simulink model "CODRTIV_v2_SystemContext"  (R2026a)
settings: Solver=VariableStepAuto
settings Model: Creator=pwilliam  LastModifiedBy=pwilliam

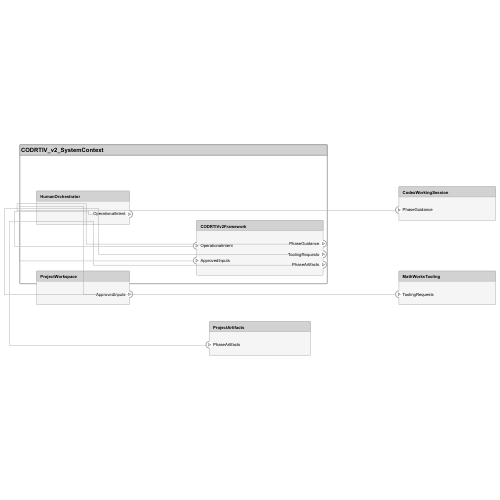
[thumbnail: Simulink's stored preview of the top-level diagram]
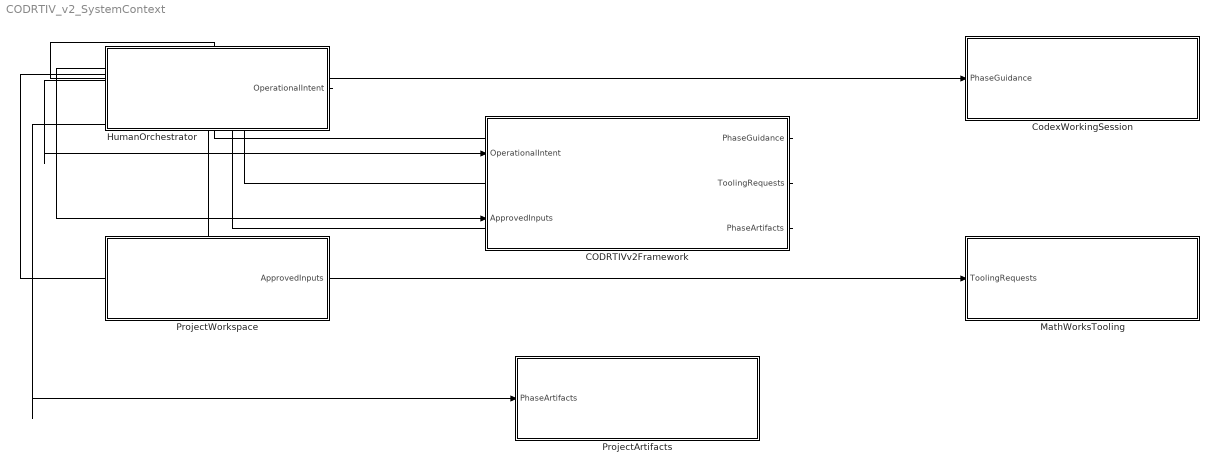
== system CODRTIV_v2_SystemContext ==
  CODRTIVv2Framework : Subsystem
      settings: PortSchema="{\"entries\":[{\"content\":{\"headerSize\":26,\"margin\":15,\"minimumSpacing\":25,\"sides\":[{\"content\":{\"connectorIds\":[\"In1\",\"In2\"]},\"type\":\"ConnectorPlacement.EquallySpacedRectSide\",\"uuid\":\"d8a99cda-410f-444c-a2c0-34a0f9144019\"},{\"content\":{\"connectorIds\":[\"Out1\",\"Out2\",\"Out3\"],\"side\":\"RIGHT\"},\"type\":\"ConnectorPlacement.EquallySpacedRectSide\",\"uuid\":\"6fbfd3a0-bc9b-423f-a970-aec3e1e13485\"},{\"content\":{\"side\":\"TOP\"},\"type\":\"ConnectorPlacement.EquallySpacedRectSide\",\"uuid\":\"0cbf1f34-d469-4804-b698-a8f91b09beec\"}]},\"type\":\"ConnectorPlacement.EquallySpacedConnector\",\"uuid\":\"a084b8e2-295c-4f11-89a7-efdb21efd295\"}],\"packageUris\":[\"http://schema.mathworks.com/mf0/Connector/R2020b\"],\"version\":\"1.0\"}"
  CodexWorkingSession : Subsystem
      settings: PortSchema="{\"entries\":[{\"content\":{\"headerSize\":26,\"margin\":15,\"minimumSpacing\":25,\"sides\":[{\"content\":{\"connectorIds\":[\"In1\"]},\"type\":\"ConnectorPlacement.EquallySpacedRectSide\",\"uuid\":\"d8a99cda-410f-444c-a2c0-34a0f9144019\"},{\"content\":{\"side\":\"RIGHT\"},\"type\":\"ConnectorPlacement.EquallySpacedRectSide\",\"uuid\":\"6fbfd3a0-bc9b-423f-a970-aec3e1e13485\"},{\"content\":{\"side\":\"TOP\"},\"type\":\"ConnectorPlacement.EquallySpacedRectSide\",\"uuid\":\"0cbf1f34-d469-4804-b698-a8f91b09beec\"}]},\"type\":\"ConnectorPlacement.EquallySpacedConnector\",\"uuid\":\"a084b8e2-295c-4f11-89a7-efdb21efd295\"}],\"packageUris\":[\"http://schema.mathworks.com/mf0/Connector/R2020b\"],\"version\":\"1.0\"}"
  HumanOrchestrator : Subsystem
      settings: PortSchema="{\"entries\":[{\"content\":{\"headerSize\":26,\"margin\":15,\"minimumSpacing\":25,\"sides\":[{\"content\":{},\"type\":\"ConnectorPlacement.EquallySpacedRectSide\",\"uuid\":\"d8a99cda-410f-444c-a2c0-34a0f9144019\"},{\"content\":{\"connectorIds\":[\"Out1\"],\"side\":\"RIGHT\"},\"type\":\"ConnectorPlacement.EquallySpacedRectSide\",\"uuid\":\"6fbfd3a0-bc9b-423f-a970-aec3e1e13485\"},{\"content\":{\"side\":\"TOP\"},\"type\":\"ConnectorPlacement.EquallySpacedRectSide\",\"uuid\":\"0cbf1f34-d469-4804-b698-a8f91b09beec\"}]},\"type\":\"ConnectorPlacement.EquallySpacedConnector\",\"uuid\":\"a084b8e2-295c-4f11-89a7-efdb21efd295\"}],\"packageUris\":[\"http://schema.mathworks.com/mf0/Connector/R2020b\"],\"version\":\"1.0\"}"
  MathWorksTooling : Subsystem
      settings: PortSchema="{\"entries\":[{\"content\":{\"headerSize\":26,\"margin\":15,\"minimumSpacing\":25,\"sides\":[{\"content\":{\"connectorIds\":[\"In1\"]},\"type\":\"ConnectorPlacement.EquallySpacedRectSide\",\"uuid\":\"d8a99cda-410f-444c-a2c0-34a0f9144019\"},{\"content\":{\"side\":\"RIGHT\"},\"type\":\"ConnectorPlacement.EquallySpacedRectSide\",\"uuid\":\"6fbfd3a0-bc9b-423f-a970-aec3e1e13485\"},{\"content\":{\"side\":\"TOP\"},\"type\":\"ConnectorPlacement.EquallySpacedRectSide\",\"uuid\":\"0cbf1f34-d469-4804-b698-a8f91b09beec\"}]},\"type\":\"ConnectorPlacement.EquallySpacedConnector\",\"uuid\":\"a084b8e2-295c-4f11-89a7-efdb21efd295\"}],\"packageUris\":[\"http://schema.mathworks.com/mf0/Connector/R2020b\"],\"version\":\"1.0\"}"
  ProjectArtifacts : Subsystem
      settings: PortSchema="{\"entries\":[{\"content\":{\"headerSize\":26,\"margin\":15,\"minimumSpacing\":25,\"sides\":[{\"content\":{\"connectorIds\":[\"In1\"]},\"type\":\"ConnectorPlacement.EquallySpacedRectSide\",\"uuid\":\"d8a99cda-410f-444c-a2c0-34a0f9144019\"},{\"content\":{\"side\":\"RIGHT\"},\"type\":\"ConnectorPlacement.EquallySpacedRectSide\",\"uuid\":\"6fbfd3a0-bc9b-423f-a970-aec3e1e13485\"},{\"content\":{\"side\":\"TOP\"},\"type\":\"ConnectorPlacement.EquallySpacedRectSide\",\"uuid\":\"0cbf1f34-d469-4804-b698-a8f91b09beec\"}]},\"type\":\"ConnectorPlacement.EquallySpacedConnector\",\"uuid\":\"a084b8e2-295c-4f11-89a7-efdb21efd295\"}],\"packageUris\":[\"http://schema.mathworks.com/mf0/Connector/R2020b\"],\"version\":\"1.0\"}"
  ProjectWorkspace : Subsystem
      settings: PortSchema="{\"entries\":[{\"content\":{\"headerSize\":26,\"margin\":15,\"minimumSpacing\":25,\"sides\":[{\"content\":{},\"type\":\"ConnectorPlacement.EquallySpacedRectSide\",\"uuid\":\"d8a99cda-410f-444c-a2c0-34a0f9144019\"},{\"content\":{\"connectorIds\":[\"Out1\"],\"side\":\"RIGHT\"},\"type\":\"ConnectorPlacement.EquallySpacedRectSide\",\"uuid\":\"6fbfd3a0-bc9b-423f-a970-aec3e1e13485\"},{\"content\":{\"side\":\"TOP\"},\"type\":\"ConnectorPlacement.EquallySpacedRectSide\",\"uuid\":\"0cbf1f34-d469-4804-b698-a8f91b09beec\"}]},\"type\":\"ConnectorPlacement.EquallySpacedConnector\",\"uuid\":\"a084b8e2-295c-4f11-89a7-efdb21efd295\"}],\"packageUris\":[\"http://schema.mathworks.com/mf0/Connector/R2020b\"],\"version\":\"1.0\"}"
  wires:
  HumanOrchestrator/1(OperationalIntent) -> CODRTIVv2Framework/1(OperationalIntent)
  ProjectWorkspace/1(ApprovedInputs) -> CODRTIVv2Framework/2(ApprovedInputs)
  CODRTIVv2Framework/1(PhaseGuidance) -> CodexWorkingSession/1(PhaseGuidance)
  CODRTIVv2Framework/2(ToolingRequests) -> MathWorksTooling/1(ToolingRequests)
  CODRTIVv2Framework/3(PhaseArtifacts) -> ProjectArtifacts/1(PhaseArtifacts)

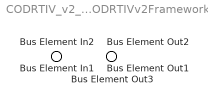
== system CODRTIV_v2_SystemContext/CODRTIVv2Framework ==
  Bus Element In1 : Inport  PortName=OperationalIntent
  Bus Element In2 : Inport  Port=2  PortName=ApprovedInputs
  Bus Element Out1 : Outport  PortName=PhaseGuidance
  Bus Element Out2 : Outport  Port=2  PortName=ToolingRequests
  Bus Element Out3 : Outport  Port=3  PortName=PhaseArtifacts

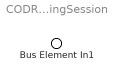
== system CODRTIV_v2_SystemContext/CodexWorkingSession ==
  Bus Element In1 : Inport  PortName=PhaseGuidance

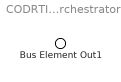
== system CODRTIV_v2_SystemContext/HumanOrchestrator ==
  Bus Element Out1 : Outport  PortName=OperationalIntent

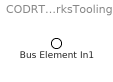
== system CODRTIV_v2_SystemContext/MathWorksTooling ==
  Bus Element In1 : Inport  PortName=ToolingRequests

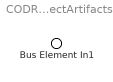
== system CODRTIV_v2_SystemContext/ProjectArtifacts ==
  Bus Element In1 : Inport  PortName=PhaseArtifacts

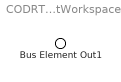
== system CODRTIV_v2_SystemContext/ProjectWorkspace ==
  Bus Element Out1 : Outport  PortName=ApprovedInputs
